simulink library "AXIDMALib"  (R2018a)
settings: Solver=ode45  StartTime=0.0  StopTime=10.0  RelTol=1e-3  EnableMultiTasking=on
undefined symbols (not defined in the file or in its folder): fftLength
libraries: simulink x4, $bdroot x4, hdlsllib x1
settings Model: Creator=mfornero  LastModifiedBy=darenlee
settings DataIOCC: LimitDataPoints=on  SaveFormat=Array
settings OptimizationCC: LifeSpan=inf
settings DebuggingCC: SolverPrmCheckMsg=warning  SFUnexpectedBacktrackingDiag=warning  SFNoUnconditionalDefaultTransitionDiag=warning  SFExecutionAtInitializationDiag=none
settings HardwareCC: ProdBitPerPointer=32  ProdBitPerSizeT=32  ProdBitPerPtrDiffT=32  ProdLargestAtomicFloat=None  ProdIntDivRoundTo=Undefined  ProdEndianess=Unspecified  ProdWordSize=32  ProdHWDeviceType=32-bit Generic
settings ModelReferenceCC: PropagateSignalLabelsOutOfModel=off
settings CodeAppCC: StateflowObjectComments=on
settings GRTTargetCC: TargetLangStandard=C89/C90 (ANSI)  GeneratePreprocessorConditionals=Disable all
settings ConfigComp: CovMetricSettings=dw  CovHtmlReporting=on  CovSaveCumulativeToWorkspaceVar=on  CovSaveSingleToWorkspaceVar=on  CovExternalEMLEnable=off  CovSFcnEnable=off

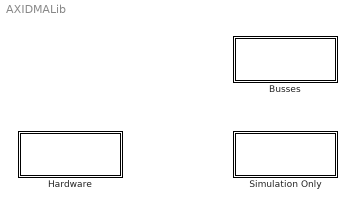
== system AXIDMALib ==
  Busses : Subsystem
  Hardware : Subsystem
  Simulation Only : Subsystem

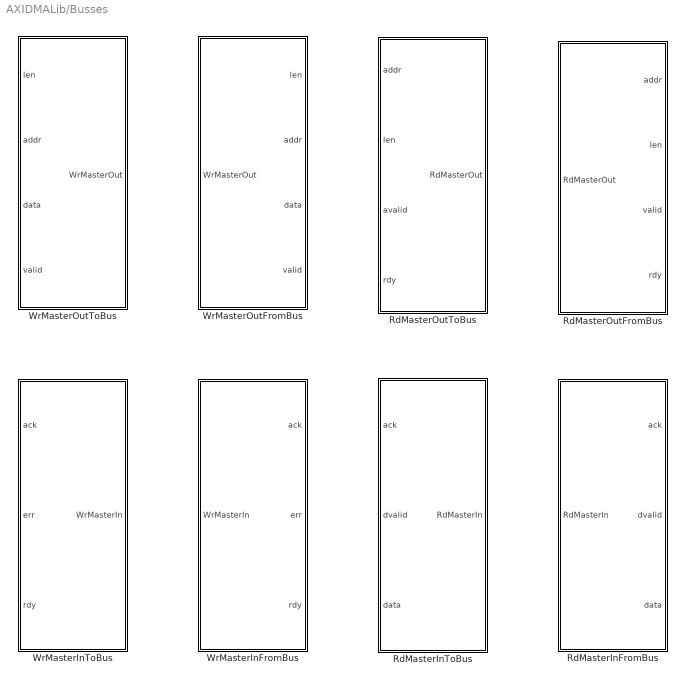
== system AXIDMALib/Busses ==
  RdMasterInFromBus : Subsystem
  RdMasterInToBus : Subsystem  mask{BusName='RdMasterInput'}
      mask prompts: BusName "Bus Name"
      mask init:
      | setupAXI4MasterBusBlock(BusName, 'Read', 'Input')
  RdMasterOutFromBus : Subsystem
  RdMasterOutToBus : Subsystem  mask{BusName='RdMasterOutput'}
      mask init:
      | setupAXI4MasterBusBlock(BusName, 'Read', 'Output')
  WrMasterInFromBus : Subsystem
  WrMasterInToBus : Subsystem  mask{BusName='WrMasterInput'}
      mask prompts: BusName "Bus Name"
      mask init:
      | setupAXI4MasterBusBlock(BusName, 'Write', 'Input')
  WrMasterOutFromBus : Subsystem
  WrMasterOutToBus : Subsystem  mask{BusName='WrMasterOutput'}
      mask init:
      | setupAXI4MasterBusBlock(BusName, 'Write', 'Output')

== system AXIDMALib/Hardware ==
  hdl_fwft_fifo : Subsystem  mask{FIFO_DEPTH=fftLength, AFULL_THRESH=2}
      mask prompts: FIFO_DEPTH "FIFO Depth"; AFULL_THRESH "Almost Full Threshold"
      mask init:
      | FIFO_CNT_BITS=ceil(log2(FIFO_DEPTH+1+3));

== system AXIDMALib/Simulation Only ==
  mem_sim : Subsystem  mask{MEM_DEPTH=fftLength*2, STALL_RATIO=[7 3]}
      mask prompts: MEM_DEPTH "Memory Depth"; STALL_RATIO "Ratio of active time to stalling time"

== system AXIDMALib/Busses/RdMasterInFromBus ==
  RdMasterIn : Inport
  Bus Selector1 : BusSelector  OutputSignals=ack,dvalid,data
  ack : Outport
  dvalid : Outport  Port=2
  data : Outport  Port=3
  wires:
  Bus Selector1/3 -> data/1  "<data>"
  Bus Selector1/2 -> dvalid/1  "<dvalid>"
  Bus Selector1/1 -> ack/1  "<ack>"
  RdMasterIn/1 -> Bus Selector1/1

== system AXIDMALib/Busses/RdMasterInToBus ==
  ack : Inport
  dvalid : Inport  Port=2
  data : Inport  Port=3
  BusCreator : BusCreator  Inputs='data','dvalid','ack'  OutDataTypeStr=Bus: RdMasterInput  NonVirtualBus=on
  RdMasterIn : Outport
  wires:
  dvalid/1 -> BusCreator/2  "dvalid"
  data/1 -> BusCreator/1  "data"
  ack/1 -> BusCreator/3  "ack"
  BusCreator/1 -> RdMasterIn/1

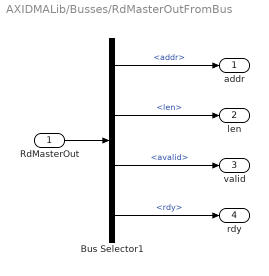
== system AXIDMALib/Busses/RdMasterOutFromBus ==
  RdMasterOut : Inport
  Bus Selector1 : BusSelector  OutputSignals=addr,len,avalid,rdy
  addr : Outport
  len : Outport  Port=2
  valid : Outport  Port=3
  rdy : Outport  Port=4
  wires:
  RdMasterOut/1 -> Bus Selector1/1
  Bus Selector1/3 -> valid/1  "<avalid>"
  Bus Selector1/2 -> len/1  "<len>"
  Bus Selector1/1 -> addr/1  "<addr>"
  Bus Selector1/4 -> rdy/1  "<rdy>"

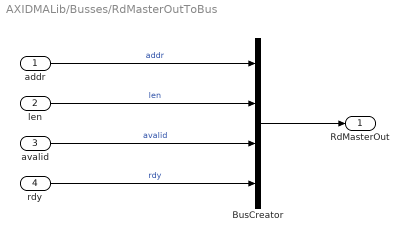
== system AXIDMALib/Busses/RdMasterOutToBus ==
  addr : Inport
  len : Inport  Port=2
  avalid : Inport  Port=3
  rdy : Inport  Port=4
  BusCreator : BusCreator  Inputs='addr','len','avalid','rdy'  OutDataTypeStr=Bus: RdMasterOutput  NonVirtualBus=on
  RdMasterOut : Outport
  wires:
  BusCreator/1 -> RdMasterOut/1
  avalid/1 -> BusCreator/3  "avalid"
  addr/1 -> BusCreator/1  "addr"
  len/1 -> BusCreator/2  "len"
  rdy/1 -> BusCreator/4  "rdy"

== system AXIDMALib/Busses/WrMasterInFromBus ==
  WrMasterIn : Inport
  Bus Selector1 : BusSelector  OutputSignals=ack,err,rdy
  ack : Outport
  err : Outport  Port=2
  rdy : Outport  Port=3
  wires:
  WrMasterIn/1 -> Bus Selector1/1
  Bus Selector1/3 -> rdy/1  "<rdy>"
  Bus Selector1/2 -> err/1  "<err>"
  Bus Selector1/1 -> ack/1  "<ack>"

== system AXIDMALib/Busses/WrMasterInToBus ==
  ack : Inport
  err : Inport  Port=2
  rdy : Inport  Port=3
  BusCreator : BusCreator  Inputs='ack','err','rdy'  OutDataTypeStr=Bus: WrMasterInput  NonVirtualBus=on
  WrMasterIn : Outport
  wires:
  BusCreator/1 -> WrMasterIn/1
  rdy/1 -> BusCreator/3  "rdy"
  ack/1 -> BusCreator/1  "ack"
  err/1 -> BusCreator/2  "err"

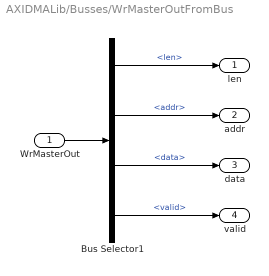
== system AXIDMALib/Busses/WrMasterOutFromBus ==
  WrMasterOut : Inport
  Bus Selector1 : BusSelector  OutputSignals=len,addr,data,valid
  len : Outport
  addr : Outport  Port=2
  data : Outport  Port=3
  valid : Outport  Port=4
  wires:
  WrMasterOut/1 -> Bus Selector1/1
  Bus Selector1/2 -> addr/1  "<addr>"
  Bus Selector1/1 -> len/1  "<len>"
  Bus Selector1/3 -> data/1  "<data>"
  Bus Selector1/4 -> valid/1  "<valid>"

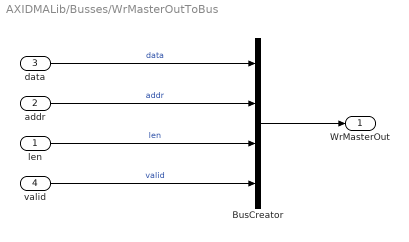
== system AXIDMALib/Busses/WrMasterOutToBus ==
  len : Inport
  addr : Inport  Port=2
  data : Inport  Port=3
  valid : Inport  Port=4
  BusCreator : BusCreator  Inputs='data','addr','len','valid'  OutDataTypeStr=Bus: WrMasterOutput  NonVirtualBus=on
  WrMasterOut : Outport
  wires:
  len/1 -> BusCreator/3  "len"
  data/1 -> BusCreator/1  "data"
  addr/1 -> BusCreator/2  "addr"
  valid/1 -> BusCreator/4  "valid"
  BusCreator/1 -> WrMasterOut/1

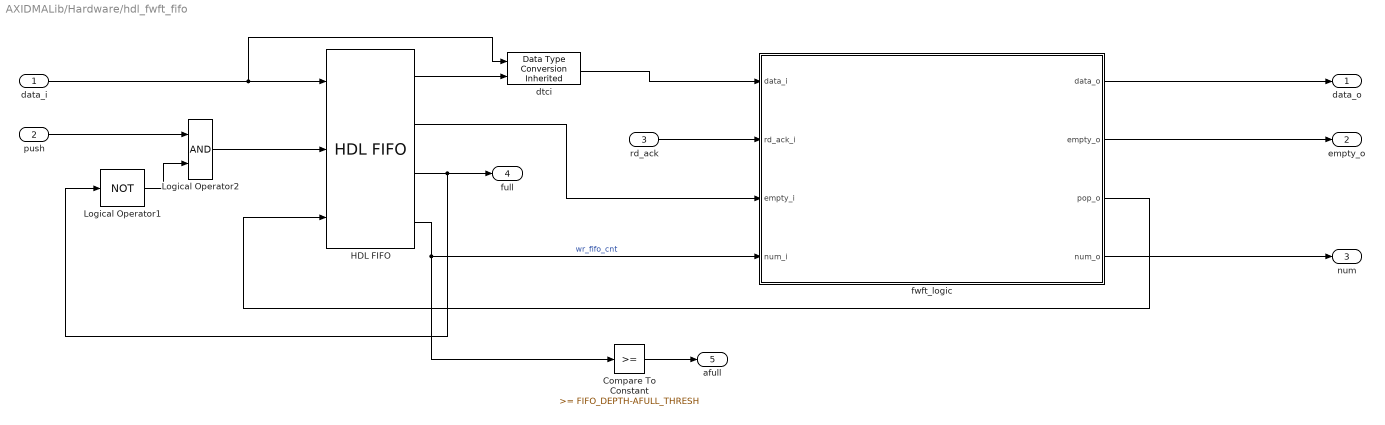
== system AXIDMALib/Hardware/hdl_fwft_fifo ==
  data_i : Inport
  push : Inport  Port=2
  rd_ack : Inport  Port=3
  Compare To Constant : simulink/Logic and Bit Operations/Compare To Constant  relop=>=  const=FIFO_DEPTH-AFULL_THRESH  OutDataTypeStr=boolean
  HDL FIFO : hdlsllib/HDL Operations/HDL FIFO  fifo_size=FIFO_DEPTH  ratio=1  push_msg=Error  pop_msg=Ignore  show_empty=on  show_full=on  show_num=on
      settings: SourceProductName=HDL Coder  SourceProductBaseCode=HD
  Logical Operator1 : Logic  Operator=NOT  IconShape=distinctive  AllPortsSameDT=off  OutDataTypeStr=boolean
  Logical Operator2 : Logic  IconShape=distinctive  AllPortsSameDT=off  OutDataTypeStr=boolean
  dtci : simulink/Signal Attributes/Data Type Conversion Inherited  ConvertRealWorld=Real World Value  DoSatur=off
      settings: SourceProductName=Simulink  SourceProductBaseCode=SL
  fwft_logic : Subsystem
  data_o : Outport
  empty_o : Outport  Port=2
  num : Outport  Port=3
  full : Outport  Port=4
  afull : Outport  Port=5
  wires:
  Compare To Constant/1 -> afull/1
  fwft_logic/1(data_o) -> data_o/1
  HDL FIFO/2 -> fwft_logic/3(empty_i)
  rd_ack/1 -> fwft_logic/2(rd_ack_i)
  fwft_logic/2(empty_o) -> empty_o/1
  data_i/1 -> dtci/1, HDL FIFO/1
  fwft_logic/3(pop_o) -> HDL FIFO/3
  push/1 -> Logical Operator2/1
  Logical Operator2/1 -> HDL FIFO/2
  Logical Operator1/1 -> Logical Operator2/2
  HDL FIFO/1 -> dtci/2
  dtci/1 -> fwft_logic/1(data_i)
  HDL FIFO/3 -> Logical Operator1/1, full/1
  HDL FIFO/4 -> Compare To Constant/1, fwft_logic/4(num_i)  "wr_fifo_cnt"
  fwft_logic/4(num_o) -> num/1

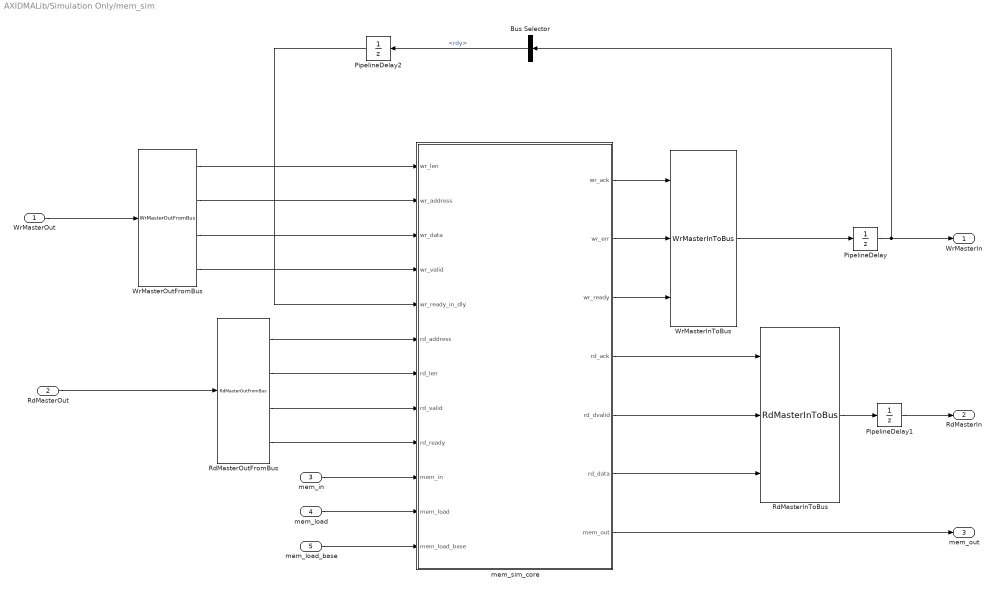
== system AXIDMALib/Simulation Only/mem_sim ==
  WrMasterOut : Inport
  RdMasterOut : Inport  Port=2
  mem_in : Inport  Port=3
  mem_load : Inport  Port=4
  mem_load_base : Inport  Port=5
  Bus Selector : BusSelector  OutputSignals=rdy
  PipelineDelay : UnitDelay  SampleTime=-1
  PipelineDelay1 : UnitDelay  SampleTime=-1
  PipelineDelay2 : UnitDelay  SampleTime=-1
  RdMasterInToBus : $bdroot/Busses/RdMasterInToBus  BusName='RdMasterInput'
  RdMasterOutFromBus : $bdroot/Busses/RdMasterOutFromBus  SystemSampleTime=-1
  WrMasterInToBus : $bdroot/Busses/WrMasterInToBus  BusName='WrMasterInput'
  WrMasterOutFromBus : $bdroot/Busses/WrMasterOutFromBus  SystemSampleTime=-1
  mem_sim_core : MATLAB Function
  WrMasterIn : Outport
  RdMasterIn : Outport  Port=2
  mem_out : Outport  Port=3
  wires:
  mem_sim_core/6(rd_data) -> RdMasterInToBus/3
  mem_sim_core/5(rd_dvalid) -> RdMasterInToBus/2
  mem_sim_core/4(rd_ack) -> RdMasterInToBus/1
  WrMasterOutFromBus/2 -> mem_sim_core/2(wr_address)
  mem_in/1 -> mem_sim_core/10(mem_in)
  RdMasterOut/1 -> RdMasterOutFromBus/1
  WrMasterOutFromBus/1 -> mem_sim_core/1(wr_len)
  mem_sim_core/3(wr_ready) -> WrMasterInToBus/3
  mem_sim_core/2(wr_err) -> WrMasterInToBus/2
  RdMasterInToBus/1 -> PipelineDelay1/1
  WrMasterOutFromBus/4 -> mem_sim_core/4(wr_valid)
  WrMasterOutFromBus/3 -> mem_sim_core/3(wr_data)
  WrMasterOut/1 -> WrMasterOutFromBus/1
  mem_sim_core/7(mem_out) -> mem_out/1
  mem_sim_core/1(wr_ack) -> WrMasterInToBus/1
  RdMasterOutFromBus/3 -> mem_sim_core/8(rd_valid)
  RdMasterOutFromBus/2 -> mem_sim_core/7(rd_len)
  RdMasterOutFromBus/1 -> mem_sim_core/6(rd_address)
  RdMasterOutFromBus/4 -> mem_sim_core/9(rd_ready)
  mem_load/1 -> mem_sim_core/11(mem_load)
  mem_load_base/1 -> mem_sim_core/12(mem_load_base)
  WrMasterInToBus/1 -> PipelineDelay/1
  PipelineDelay1/1 -> RdMasterIn/1
  PipelineDelay2/1 -> mem_sim_core/5(wr_ready_in_dly)
  PipelineDelay/1 -> Bus Selector/1, WrMasterIn/1
  Bus Selector/1 -> PipelineDelay2/1  "<rdy>"

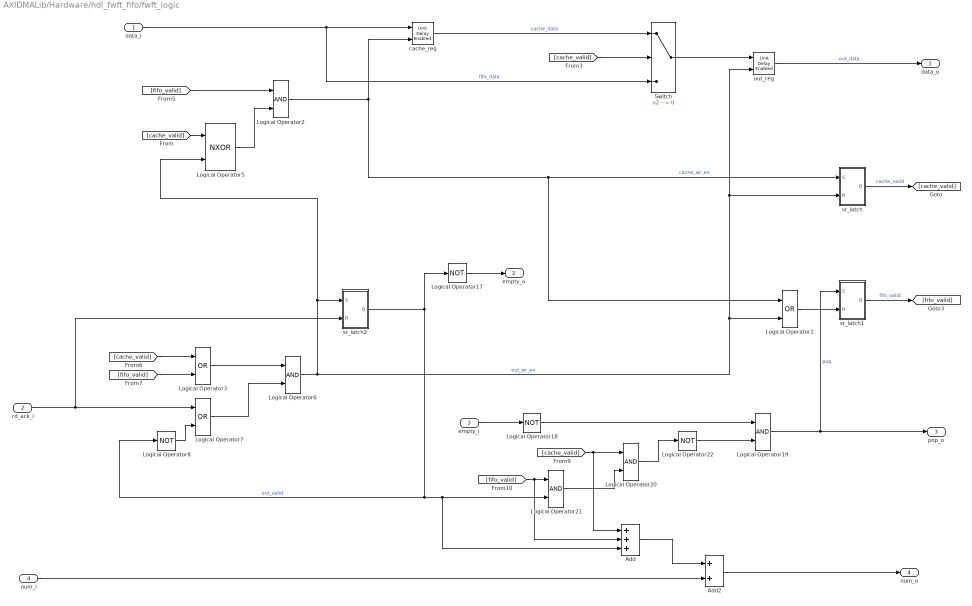
== system AXIDMALib/Hardware/hdl_fwft_fifo/fwft_logic ==
  data_i : Inport
  rd_ack_i : Inport  Port=2
  empty_i : Inport  Port=3
  num_i : Inport  Port=4
  Add : Sum  Inputs=+++  AccumDataTypeStr=fixdt(0,2,0)
  Add2 : Sum  OutDataTypeStr=fixdt(0,FIFO_CNT_BITS,0)
  Logical Operator1 : Logic  Operator=OR  IconShape=distinctive  AllPortsSameDT=off  OutDataTypeStr=boolean
  Logical Operator{8,17..18,22} (4 alike) : Logic  Operator=NOT  IconShape=distinctive  AllPortsSameDT=off  OutDataTypeStr=boolean
  Logical Operator{2,6,19..21} (5 alike) : Logic  IconShape=distinctive  AllPortsSameDT=off  OutDataTypeStr=boolean
  Logical Operator3 : Logic  Operator=OR  IconShape=distinctive  AllPortsSameDT=off  OutDataTypeStr=boolean
  Logical Operator5 : Logic  Operator=NXOR  IconShape=distinctive  AllPortsSameDT=off  OutDataTypeStr=boolean
  Logical Operator7 : Logic  Operator=OR  IconShape=distinctive  AllPortsSameDT=off  OutDataTypeStr=boolean
  Switch : Switch  Criteria=u2 ~= 0
  cache_reg : simulink/Additional Math & Discrete/Additional Discrete/Unit Delay Enabled  vinit=0.0  tsamp=-1
      settings: SourceProductName=Simulink  SourceProductBaseCode=SL
  out_reg : simulink/Additional Math & Discrete/Additional Discrete/Unit Delay Enabled  vinit=0.0  tsamp=-1
      settings: SourceProductName=Simulink  SourceProductBaseCode=SL
  sr_latch : Subsystem
  sr_latch1 : Subsystem
  sr_latch2 : Subsystem
  data_o : Outport
  empty_o : Outport  Port=2
  pop_o : Outport  Port=3
  num_o : Outport  Port=4
  wires:
  empty_i/1 -> Logical Operator18/1
  sr_latch1/1(Q) -> [fifo_valid]  "fifo_valid"
  sr_latch/1(Q) -> [cache_valid]  "cache_valid"
  Switch/1 -> out_reg/1
  data_i/1 -> Switch/3, cache_reg/1  "fifo_data"
  cache_reg/1 -> Switch/1  "cache_data"
  Logical Operator5/1 -> Logical Operator2/2
  Logical Operator6/1 -> Logical Operator5/2, sr_latch2/1(S), out_reg/2, sr_latch/2(R), Logical Operator1/2  "out_wr_en"
  [cache_valid] -> Logical Operator5/1
  [cache_valid] -> Switch/2
  Logical Operator2/1 -> cache_reg/2, Logical Operator1/1, sr_latch/1(S)  "cache_wr_en"
  [fifo_valid] -> Logical Operator2/1
  [cache_valid] -> Logical Operator3/1
  [fifo_valid] -> Logical Operator3/2
  Logical Operator3/1 -> Logical Operator6/1
  Logical Operator7/1 -> Logical Operator6/2
  rd_ack_i/1 -> sr_latch2/2(R), Logical Operator7/1
  sr_latch2/1(Q) -> Logical Operator8/1, Add/3, Logical Operator21/2, Logical Operator17/1  "out_valid"
  Logical Operator8/1 -> Logical Operator7/2
  Logical Operator17/1 -> empty_o/1
  Logical Operator18/1 -> Logical Operator19/1
  Logical Operator21/1 -> Logical Operator20/2
  Logical Operator22/1 -> Logical Operator19/2
  Logical Operator20/1 -> Logical Operator22/1
  Logical Operator19/1 -> pop_o/1, sr_latch1/1(S)  "pop"
  [cache_valid] -> Add/1, Logical Operator20/1
  [fifo_valid] -> Add/2, Logical Operator21/1
  Logical Operator1/1 -> sr_latch1/2(R)
  out_reg/1 -> data_o/1  "out_data"
  num_i/1 -> Add2/2
  Add/1 -> Add2/1
  Add2/1 -> num_o/1

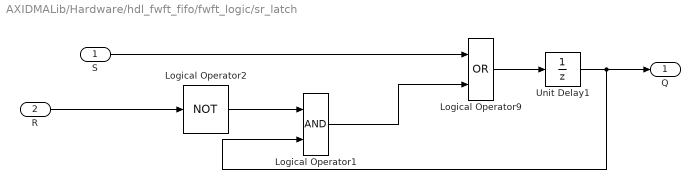
== system AXIDMALib/Hardware/hdl_fwft_fifo/fwft_logic/sr_latch ==
  S : Inport
  R : Inport  Port=2
  Logical Operator1 : Logic  IconShape=distinctive  AllPortsSameDT=off  OutDataTypeStr=boolean
  Logical Operator2 : Logic  Operator=NOT  IconShape=distinctive  AllPortsSameDT=off  OutDataTypeStr=boolean
  Logical Operator9 : Logic  Operator=OR  IconShape=distinctive  AllPortsSameDT=off  OutDataTypeStr=boolean
  Unit Delay1 : UnitDelay  SampleTime=-1
  Q : Outport
  wires:
  S/1 -> Logical Operator9/1
  R/1 -> Logical Operator2/1
  Logical Operator2/1 -> Logical Operator1/1
  Unit Delay1/1 -> Logical Operator1/2, Q/1
  Logical Operator9/1 -> Unit Delay1/1
  Logical Operator1/1 -> Logical Operator9/2

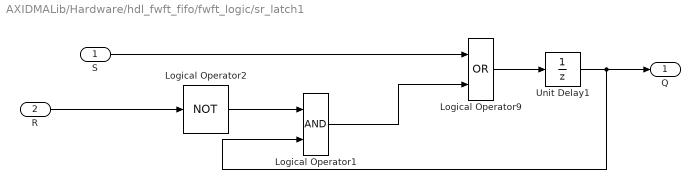
== system AXIDMALib/Hardware/hdl_fwft_fifo/fwft_logic/sr_latch1 ==
  S : Inport
  R : Inport  Port=2
  Logical Operator1 : Logic  IconShape=distinctive  AllPortsSameDT=off  OutDataTypeStr=boolean
  Logical Operator2 : Logic  Operator=NOT  IconShape=distinctive  AllPortsSameDT=off  OutDataTypeStr=boolean
  Logical Operator9 : Logic  Operator=OR  IconShape=distinctive  AllPortsSameDT=off  OutDataTypeStr=boolean
  Unit Delay1 : UnitDelay  SampleTime=-1
  Q : Outport
  wires:
  Logical Operator1/1 -> Logical Operator9/2
  Logical Operator9/1 -> Unit Delay1/1
  Unit Delay1/1 -> Q/1, Logical Operator1/2
  Logical Operator2/1 -> Logical Operator1/1
  R/1 -> Logical Operator2/1
  S/1 -> Logical Operator9/1

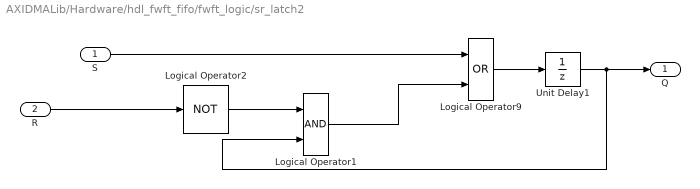
== system AXIDMALib/Hardware/hdl_fwft_fifo/fwft_logic/sr_latch2 ==
  S : Inport
  R : Inport  Port=2
  Logical Operator1 : Logic  IconShape=distinctive  AllPortsSameDT=off  OutDataTypeStr=boolean
  Logical Operator2 : Logic  Operator=NOT  IconShape=distinctive  AllPortsSameDT=off  OutDataTypeStr=boolean
  Logical Operator9 : Logic  Operator=OR  IconShape=distinctive  AllPortsSameDT=off  OutDataTypeStr=boolean
  Unit Delay1 : UnitDelay  SampleTime=-1
  Q : Outport
  wires:
  S/1 -> Logical Operator9/1
  R/1 -> Logical Operator2/1
  Logical Operator2/1 -> Logical Operator1/1
  Unit Delay1/1 -> Logical Operator1/2, Q/1
  Logical Operator9/1 -> Unit Delay1/1
  Logical Operator1/1 -> Logical Operator9/2

== matlab function AXIDMALib/Simulation Only/mem_sim/mem_sim_core ==
  data: wr_len input; wr_ack output; wr_err output; wr_address input; wr_data input; wr_valid input; wr_ready_in_dly input boolean; rd_address input; rd_len input; rd_valid input; rd_ready input; mem_in input; wr_ready output; rd_ack output; rd_dvalid output; rd_data output; mem_out output; mem_load input; mem_load_base input; MEM_DEPTH parameter; STALL_RATIO parameter
function [wr_ack, wr_err, wr_ready, rd_ack, rd_dvalid, rd_data, mem_out] = ...
    mem_sim(wr_len, wr_address, wr_data, wr_valid, wr_ready_in_dly, rd_address, rd_len, rd_valid, rd_ready,...
            mem_in, mem_load, mem_load_base, MEM_DEPTH, STALL_RATIO)
%#codegen

STATE_IDLE = 0;
STATE_ACTIVE = 1;
STATE_STALL = 2;
STATE_WAIT = 3;

NT_WDATA = numerictype(fi(wr_data));
NT_RDATA = numerictype(fi(mem_in));

persistent wrstate rdstate mem wr_addr wr_cnt rd_addr rd_cnt wr_stall_cnt
if isempty(wrstate)
    wr_stall_cnt = 0;
    wrstate = STATE_IDLE;
    rdstate = STATE_IDLE;
    mem = zeros(MEM_DEPTH,1,'like', fi(wr_data));
    wr_addr = zeros(1,1, 'like', wr_address);
    wr_cnt = zeros(1,1, 'like', wr_len);
    rd_cnt = zeros(1,1, 'like', rd_len);
    rd_addr = zeros(1,1, 'like', rd_address);
end

wr_ack = false;
wr_ready = false;
wr_err = false;
rd_ack = false;
rd_dvalid = false;
rd_data = zeros(1,1, 'like', fi(mem_in));
mem_out = mem;

rd_rdy = logical(rd_ready);

num_wr_bytes = 2^ceil(log2(ceil(NT_WDATA.WordLength / 8)));
wr_word_addr = double(wr_address) / num_wr_bytes;

num_rd_bytes = 2^ceil(log2(ceil(NT_RDATA.WordLength / 8)));
rd_word_addr = double(rd_address) / num_rd_bytes;

load_word_addr = double(mem_load_base) / num_rd_bytes;


switch rdstate
    case STATE_IDLE
        if rd_valid
            rd_cnt(:) = rd_len-1;
            rdstate = STATE_ACTIVE;
            rd_addr(:) = rd_word_addr;
        end
    case STATE_ACTIVE
        if rd_cnt == 0
            rdstate = STATE_WAIT;
        elseif ~rd_rdy
            rdstate = STATE_STALL;
        end
        rd_addr(:) = rd_addr + 1;    
        rd_cnt(:) = rd_cnt - 1;
        rd_dvalid = true;
    case STATE_STALL
        if rd_rdy
            rdstate = STATE_ACTIVE;
        end
    case STATE_WAIT
        if rd_cnt == 3
            rd_ack = true;
            rdstate = STATE_IDLE;
        else
            rd_cnt(:) = rd_cnt + 1;
        end
end

rd_data(:) = mem(max(1,rd_addr));

switch wrstate
    case STATE_IDLE
        if wr_valid
            wr_cnt(:) =  wr_len-1;
            wrstate = STATE_ACTIVE;
            wr_addr(:) = wr_word_addr;
            wr_stall_cnt = STALL_RATIO(1);
        end
        wr_ready = true;
    case STATE_ACTIVE
        if wr_cnt == 0
            wrstate = STATE_WAIT;
            wr_ready = false;
        else
            if wr_valid
                wr_addr(:) = wr_addr + 1;    
                wr_cnt(:) =  wr_cnt - 1;
            end
            if wr_stall_cnt == 0 && STALL_RATIO(2) > 0
                wrstate = STATE_STALL;
                wr_stall_cnt = STALL_RATIO(2);
                wr_ready = false;
            else
                wr_stall_cnt = wr_stall_cnt -1;
                wr_ready = true;
            end
        end
    case STATE_STALL
        if wr_cnt == 0
            wrstate = STATE_WAIT;
        elseif wr_stall_cnt == 0
            wrstate = STATE_ACTIVE;
            wr_stall_cnt = STALL_RATIO(1);
        else
            wr_stall_cnt = wr_stall_cnt -1;
        end
        wr_ready = false;
        if wr_valid && wr_ready_in_dly
            wr_addr(:) = wr_addr + 1;    
            wr_cnt(:) =  wr_cnt - 1;
        elseif wr_valid
            error('Attempting to write data while ready is low');
        end
    case STATE_WAIT
        wr_ready = false;
        if wr_cnt == 3
            wr_ack = true;
            wrstate = STATE_IDLE;
        else
            wr_cnt(:) = wr_cnt + 1;
        end
        
end

if wr_valid
    mem(wr_addr+1) = wr_data;
end

if mem_load
    mem(load_word_addr+1:numel(mem_in)) = mem_in;
end
